simulink model "starterProject02"  (R2020b)
settings: Solver=ode1  StartTime=0.0  StopTime=inf  FixedStep=0.001  RelTol=1e-3  EnableMultiTasking=on
libraries: arduinolib x4
settings Model: DataDictionary=arduinoProject02DD.sldd  FPTRunName=Active  SILPILModeSetting=veronly  ExtModeTrigDuration=2  Creator=kitaw  LastModifiedBy=kitaw
settings DataIOCC: LimitDataPoints=on  SaveFormat=Array
settings OptimizationCC: ExpressionDepthLimit=2147483647  LifeSpan=Inf  MaxStackSize=64
settings DebuggingCC: UnderspecifiedInitializationDetection=Classic  MergeDetectMultiDrivingBlocksExec=none  FcnCallInpInsideContextMsg=warning  AllowSymbolicDim=off  StateNameClashWarn=warning  SFUnexpectedBacktrackingDiag=warning  SFNoUnconditionalDefaultTransitionDiag=warning  SFExecutionAtInitializationDiag=none  ArithmeticOperatorsInVariantConditions=warning
settings HardwareCC: ProdBitPerInt=16  ProdBitPerPointer=16  ProdBitPerSizeT=16  ProdBitPerPtrDiffT=16  ProdLargestAtomicFloat=None  ProdWordSize=8  ProdHWDeviceType=Atmel->AVR  UseEmbeddedCoderFeatures=off  UseSimulinkCoderFeatures=off
settings ModelReferenceCC: PropagateSignalLabelsOutOfModel=off
settings SFSimCC: SimUseLocalCustomCode=off  CustomCodeUndefinedFunction=UseInterfaceOnly
settings RTWCC: Description=Embedded Coder  SystemTargetFile=ert.tlc  HardwareBoard=Arduino Uno  TemplateMakefile=ert_default_tmf  GenerateReport=on  RTWVerbose=off  RTWUseLocalCustomCode=off  Toolchain=Arduino AVR  BuildConfiguration=Faster Runs  LaunchReport=on
settings CodeAppCC: ForceParamTrailComments=on  OperatorAnnotations=on  StateflowObjectComments=on  MATLABSourceComments=on
settings ERTTargetCC: MultiwordLength=2048  ERTCustomFileBanners=off  SupportContinuousTime=on  SupportNonInlinedSFcns=on  RemoveResetFunc=off  SupportVariableSizeSignals=on  ModelStepFunctionPrototypeControlCompliant=off  ExtModeStaticAllocSize=250
settings ConfigComp: CovMetricSettings=dw  CovSaveCumulativeToWorkspaceVar=on  CovSaveSingleToWorkspaceVar=on  CovExternalEMLEnable=off  CovSFcnEnable=off

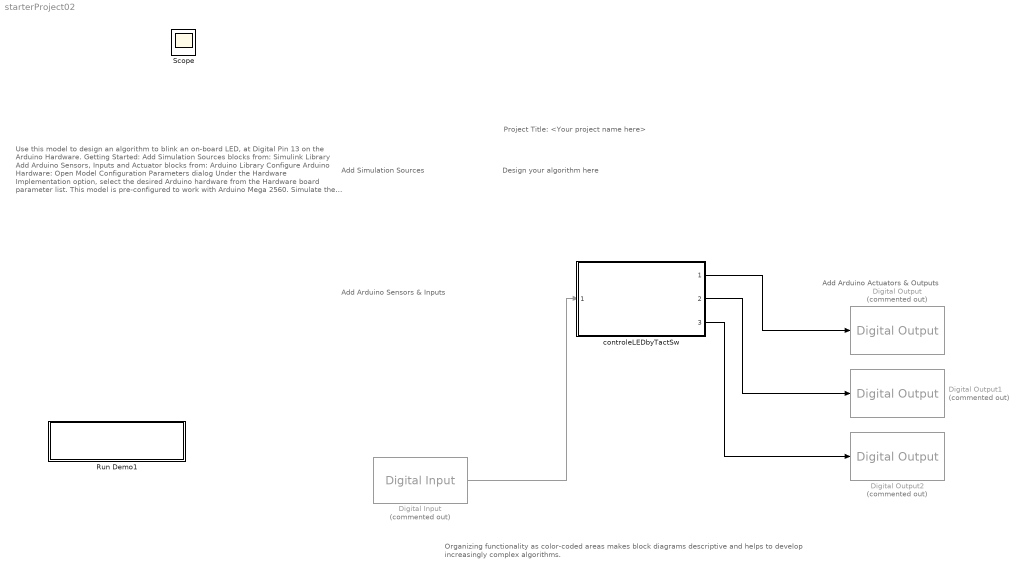
== system starterProject02 ==
  note: Organizing functionality as color-coded areas makes block diagrams descriptive and helps to develop increasingly complex algorithms.
  note: Add Arduino Actuators & Outputs
  note: Use this model to design an algorithm to blink an on-board LED, at Digital Pin 13 on the Arduino Hardware.
      |
      | Getting Started:
      |
      | Add Simulation Sources blocks from:
      | Simulink Library
      | Add Arduino Sensors, Inputs and Actuator blocks from:
      | Arduino Library
      |
      | Configure Arduino Hardware:
      |
      | Open Model Configuration Parameters dialog
      | Under the Hardware Implementation option, select the desired Arduino hardware from the Hardware board parameter list.
      |
      | This model is pre-configured to work with Arduino Mega 2560.
      |
      | Simulate the Model
      |
      | Click the Run button on the Simulink Editor toolbar.
      |
      | Run the Model on Arduino Hardware
      |
      | Click the Deploy to Hardware button on the Simulink Editor toolbar.
      |
      | Other Things to Try:
      |
      | Create and run a model that repeatedly brightens and dims an LED. Hint: Use PWM block as an Arduino actuator.
  note: Add Arduino Sensors & Inputs
  note: Design your algorithm here
  note: Add Simulation Sources
  note: Project Title: <Your project name here>
  Digital Input : arduinolib/Digital Input  Commented=on  pinNumber=2  mode=Default  Direction=input  SampleTime=-1  blockPlatform=arduino
  Digital Output : arduinolib/Digital Output  Commented=on  pinNumber=3  Direction=output  blockPlatform=arduino
  Digital Output1 : arduinolib/Digital Output  Commented=on  pinNumber=4  Direction=output  blockPlatform=arduino
  Digital Output2 : arduinolib/Digital Output  Commented=on  pinNumber=5  Direction=output  blockPlatform=arduino
  Run Demo1 : Subsystem  Description=Controls host-side RTDX processing.
      mask Display: pic=imread('arduinoDeploytoHardware.png');image(pic);
  controleLEDbyTactSw : Subsystem  TreatAsAtomicUnit=on  ReferencedSubsystem=controleLEDbyTactSw
  Scope : Scope
  wires:
  Digital Input/1 -> controleLEDbyTactSw/1
  controleLEDbyTactSw/1 -> Digital Output/1
  controleLEDbyTactSw/2 -> Digital Output1/1
  controleLEDbyTactSw/3 -> Digital Output2/1

== system starterProject02/Run Demo1 ==
